simulink model "dis_try"  (Simulink 8.7)
settings: Solver=FixedStepAuto  StartTime=0.0  StopTime=10.0  RelTol=1e-3
undefined symbols (not defined in the file or in its folder): dyn_return
settings Model: Creator=Godric  LastModifiedBy=Godric
settings DataIOCC: LimitDataPoints=off  SaveFormat=Dataset
settings DebuggingCC: UnderspecifiedInitializationDetection=Simplified  MergeDetectMultiDrivingBlocksExec=error
settings HardwareCC: ProdBitPerPointer=64  ProdLargestAtomicFloat=Float  ProdIntDivRoundTo=Zero  ProdEndianess=LittleEndian  ProdWordSize=64  ProdHWDeviceType=Intel->x86-64 (Windows64)
settings ModelReferenceCC: PropagateSignalLabelsOutOfModel=on
settings ConfigComp: CovModelRefEnable=off

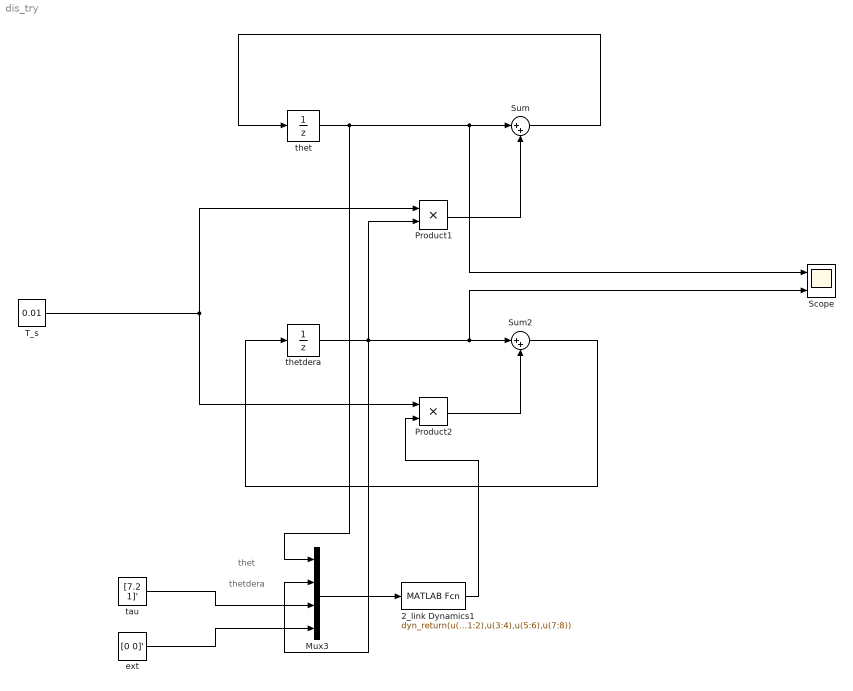
== system dis_try ==
  note: thetdera
  note: thet
  2_link Dynamics1 : MATLABFcn  MATLABFcn=dyn_return(u(1:2),u(3:4),u(5:6),u(7:8))  OutputDimensions=[2,1]  Output1D=off
  Mux3 : Mux
  Product1 : Product
  Product2 : Product
  Scope : Scope  NumInputPorts=2
  Sum : Sum  Inputs=|++
  Sum2 : Sum  Inputs=|++
  T_s : Constant  Value=0.01
  ext : Constant  Value=[0 0]'
  tau : Constant  Value=[7.2 1]'
  thet : UnitDelay  SampleTime=-1
  thetdera : UnitDelay  SampleTime=-1
  wires:
  thet/1 -> Mux3/1, Scope/1, Sum/1
  Product1/1 -> Sum/2
  T_s/1 -> Product1/1, Product2/1
  thetdera/1 -> Mux3/2, Scope/2, Sum2/1, Product1/2
  Sum/1 -> thet/1
  Product2/1 -> Sum2/2
  Sum2/1 -> thetdera/1
  Mux3/1 -> 2_link Dynamics1/1
  tau/1 -> Mux3/3
  ext/1 -> Mux3/4
  2_link Dynamics1/1 -> Product2/2
